simulink model "Simulare_cu_Ackermann"  (R2023b)
settings: Solver=VariableStepAuto  StartTime=0.0  StopTime=10  FixedStep=0.01  RelTol=1e-3
values from neighbouring files (symbols this model uses):
  K = Z/P    [LMI.m]    (also in Workspace.mat = 8.82782218537; model_simulation.m = lqr(A,B,Q,R,0.01))
  T = 0.8    [model_robust.m]
undefined symbols (not defined in the file or in its folder): L
settings Model: Creator=petri  LastModifiedBy=petri

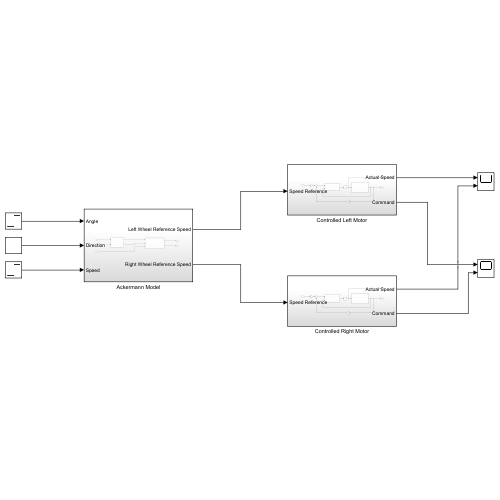
[thumbnail: Simulink's stored preview of the top-level diagram]
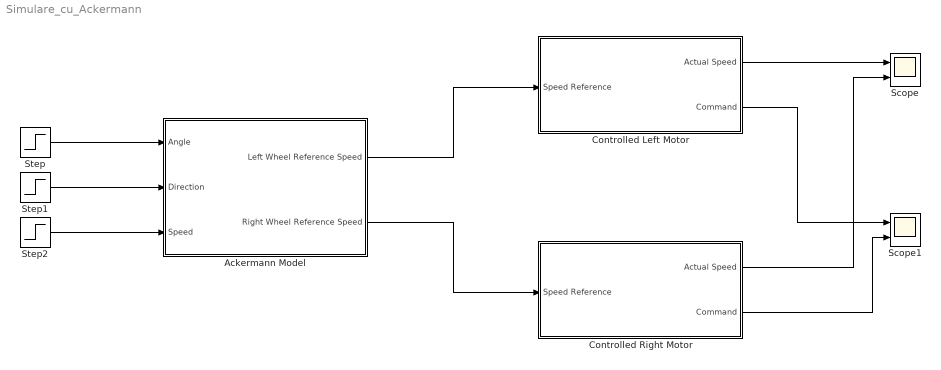
== system Simulare_cu_Ackermann ==
  Ackermann Model : Subsystem
  Controlled Left Motor : Subsystem
  Controlled Right Motor : Subsystem
  Scope : Scope  NumInputPorts=2
  Scope1 : Scope  NumInputPorts=2
  Step : Step  After=30  SampleTime=0
  Step1 : Step  SampleTime=0
  Step2 : Step  After=120  SampleTime=0
  wires:
  Ackermann Model/1(Left Wheel Reference Speed) -> Controlled Left Motor/1(Speed Reference)
  Ackermann Model/2(Right Wheel Reference Speed) -> Controlled Right Motor/1(Speed Reference)
  Step/1 -> Ackermann Model/1(Angle)
  Step1/1 -> Ackermann Model/2(Direction)
  Step2/1 -> Ackermann Model/3(Speed)
  Controlled Left Motor/1(Actual Speed) -> Scope/1
  Controlled Left Motor/2(Command) -> Scope1/1
  Controlled Right Motor/1(Actual Speed) -> Scope/2
  Controlled Right Motor/2(Command) -> Scope1/2

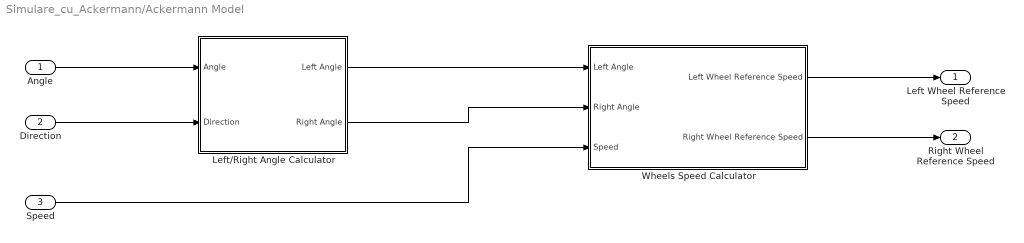
== system Simulare_cu_Ackermann/Ackermann Model ==
  Angle : Inport
  Direction : Inport  Port=2
  Speed : Inport  Port=3
  Left/Right Angle Calculator : Subsystem
  Wheels Speed Calculator : Subsystem
  Left Wheel Reference Speed : Outport
  Right Wheel Reference Speed : Outport  Port=2
  wires:
  Wheels Speed Calculator/1(Left Wheel Reference Speed) -> Left Wheel Reference Speed/1
  Left/Right Angle Calculator/2(Right Angle) -> Wheels Speed Calculator/2(Right Angle)
  Angle/1 -> Left/Right Angle Calculator/1(Angle)
  Left/Right Angle Calculator/1(Left Angle) -> Wheels Speed Calculator/1(Left Angle)
  Speed/1 -> Wheels Speed Calculator/3(Speed)
  Direction/1 -> Left/Right Angle Calculator/2(Direction)
  Wheels Speed Calculator/2(Right Wheel Reference Speed) -> Right Wheel Reference Speed/1

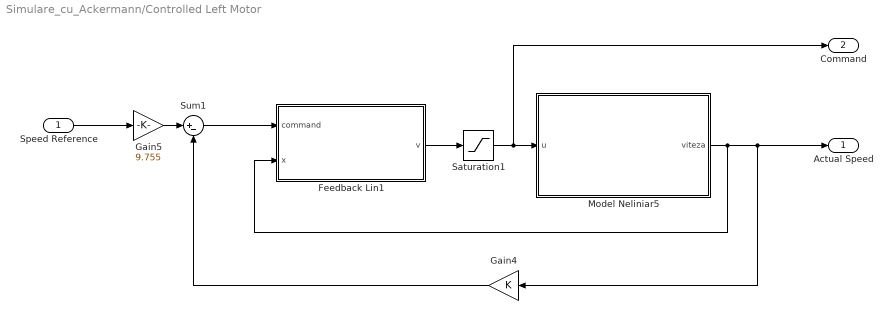
== system Simulare_cu_Ackermann/Controlled Left Motor ==
  Speed Reference : Inport
  Feedback Lin1 : Subsystem
  Gain4 : Gain  Gain=K
  Gain5 : Gain  Gain=9.755
  Model Neliniar5 : Subsystem
  Saturation1 : Saturate  UpperLimit=0.3  LowerLimit=0
  Sum1 : Sum  Inputs=|+-
  Actual Speed : Outport
  Command : Outport  Port=2
  wires:
  Speed Reference/1 -> Gain5/1
  Feedback Lin1/1(v) -> Saturation1/1
  Saturation1/1 -> Command/1, Model Neliniar5/1(u)
  Model Neliniar5/1(viteza) -> Actual Speed/1, Gain4/1, Feedback Lin1/2(x)
  Sum1/1 -> Feedback Lin1/1(command)
  Gain4/1 -> Sum1/2
  Gain5/1 -> Sum1/1

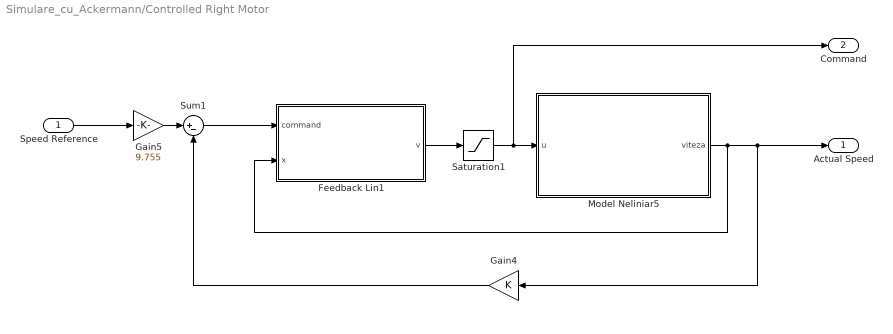
== system Simulare_cu_Ackermann/Controlled Right Motor ==
  Speed Reference : Inport
  Feedback Lin1 : Subsystem
  Gain4 : Gain  Gain=K
  Gain5 : Gain  Gain=9.755
  Model Neliniar5 : Subsystem
  Saturation1 : Saturate  UpperLimit=0.3  LowerLimit=0
  Sum1 : Sum  Inputs=|+-
  Actual Speed : Outport
  Command : Outport  Port=2
  wires:
  Speed Reference/1 -> Gain5/1
  Feedback Lin1/1(v) -> Saturation1/1
  Saturation1/1 -> Command/1, Model Neliniar5/1(u)
  Model Neliniar5/1(viteza) -> Actual Speed/1, Gain4/1, Feedback Lin1/2(x)
  Sum1/1 -> Feedback Lin1/1(command)
  Gain4/1 -> Sum1/2
  Gain5/1 -> Sum1/1

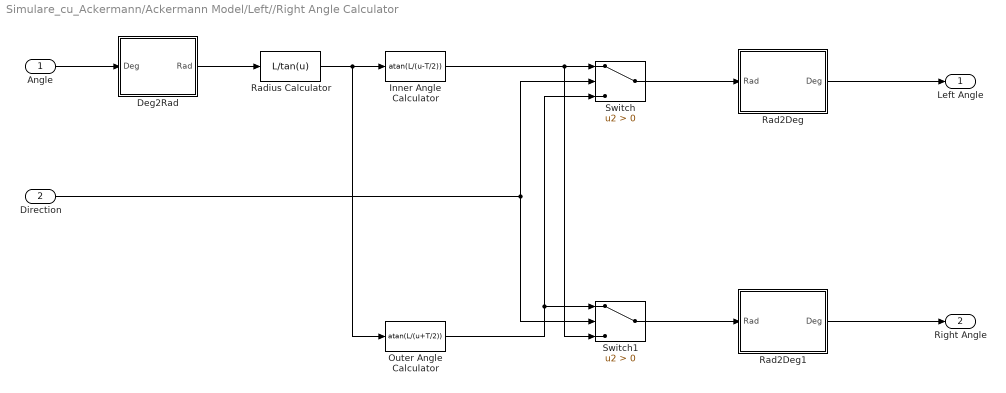
== system Simulare_cu_Ackermann/Ackermann Model/Left//Right Angle Calculator ==
  Angle : Inport
  Direction : Inport  Port=2
  Deg2Rad : Subsystem
  Inner Angle Calculator : Fcn  Expr=atan(L/(u-T/2))
  Outer Angle Calculator : Fcn  Expr=atan(L/(u+T/2))
  Rad2Deg : Subsystem
  Rad2Deg1 : Subsystem
  Radius Calculator : Fcn  Expr=L/tan(u)
  Switch : Switch  Criteria=u2 > Threshold  SaturateOnIntegerOverflow=off  InputSameDT=off
  Switch1 : Switch  Criteria=u2 > Threshold  SaturateOnIntegerOverflow=off  InputSameDT=off
  Left Angle : Outport
  Right Angle : Outport  Port=2
  wires:
  Direction/1 -> Switch/2, Switch1/2
  Angle/1 -> Deg2Rad/1(Deg)
  Outer Angle Calculator/1 -> Switch1/1, Switch/3
  Inner Angle Calculator/1 -> Switch/1, Switch1/3
  Switch/1 -> Rad2Deg/1(Rad)
  Switch1/1 -> Rad2Deg1/1(Rad)
  Rad2Deg1/1(Deg) -> Right Angle/1
  Rad2Deg/1(Deg) -> Left Angle/1
  Radius Calculator/1 -> Inner Angle Calculator/1, Outer Angle Calculator/1
  Deg2Rad/1(Rad) -> Radius Calculator/1

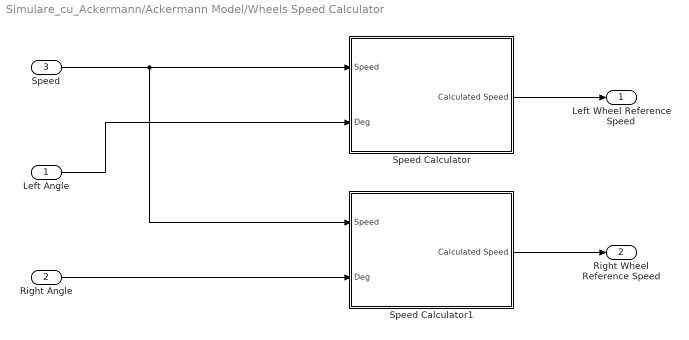
== system Simulare_cu_Ackermann/Ackermann Model/Wheels Speed Calculator ==
  Left Angle : Inport
  Right Angle : Inport  Port=2
  Speed : Inport  Port=3
  Speed Calculator : Subsystem
  Speed Calculator1 : Subsystem
  Left Wheel Reference Speed : Outport
  Right Wheel Reference Speed : Outport  Port=2
  wires:
  Speed Calculator1/1(Calculated Speed) -> Right Wheel Reference Speed/1
  Right Angle/1 -> Speed Calculator1/2(Deg)
  Speed/1 -> Speed Calculator/1(Speed), Speed Calculator1/1(Speed)
  Speed Calculator/1(Calculated Speed) -> Left Wheel Reference Speed/1
  Left Angle/1 -> Speed Calculator/2(Deg)

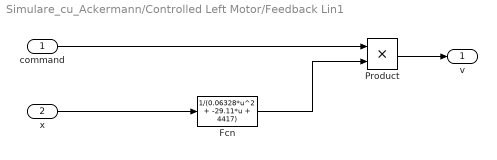
== system Simulare_cu_Ackermann/Controlled Left Motor/Feedback Lin1 ==
  command : Inport
  x : Inport  Port=2
  Fcn : Fcn  Expr=1/(0.06328*u^2 + -29.11*u + 4417)
  Product : Product
  v : Outport
  wires:
  Product/1 -> v/1
  Fcn/1 -> Product/2
  command/1 -> Product/1
  x/1 -> Fcn/1

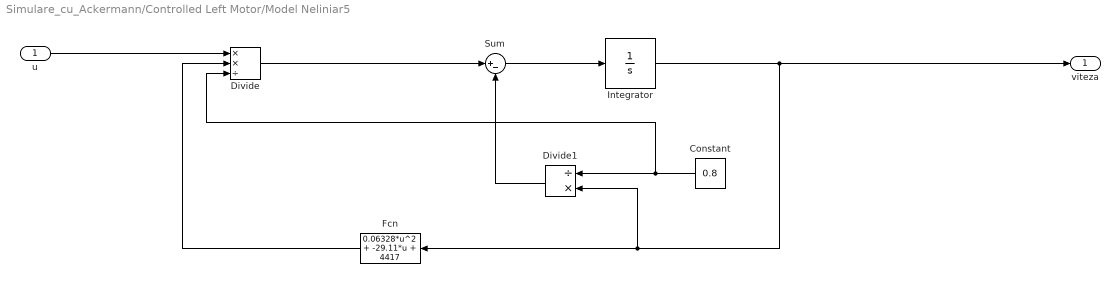
== system Simulare_cu_Ackermann/Controlled Left Motor/Model Neliniar5 ==
  u : Inport
  Constant : Constant  Value=0.8
  Divide : Product  Inputs=**/
  Divide1 : Product  Inputs=/*
  Fcn : Fcn  Expr=0.06328*u^2 + -29.11*u + 4417
  Integrator : Integrator
  Sum : Sum  Inputs=|+-
  viteza : Outport
  wires:
  u/1 -> Divide/1
  Constant/1 -> Divide1/1, Divide/3
  Integrator/1 -> viteza/1, Fcn/1, Divide1/2
  Sum/1 -> Integrator/1
  Divide1/1 -> Sum/2
  Divide/1 -> Sum/1
  Fcn/1 -> Divide/2

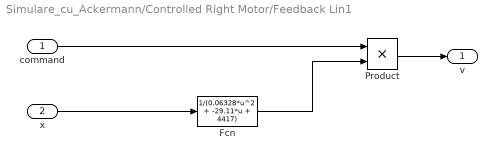
== system Simulare_cu_Ackermann/Controlled Right Motor/Feedback Lin1 ==
  command : Inport
  x : Inport  Port=2
  Fcn : Fcn  Expr=1/(0.06328*u^2 + -29.11*u + 4417)
  Product : Product
  v : Outport
  wires:
  Product/1 -> v/1
  Fcn/1 -> Product/2
  command/1 -> Product/1
  x/1 -> Fcn/1

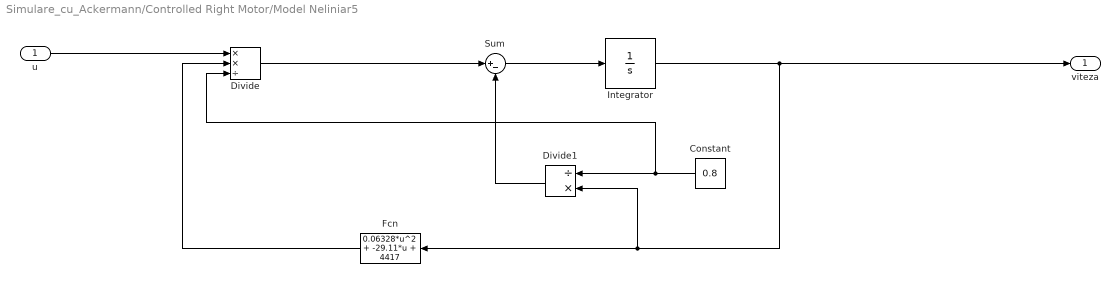
== system Simulare_cu_Ackermann/Controlled Right Motor/Model Neliniar5 ==
  u : Inport
  Constant : Constant  Value=0.8
  Divide : Product  Inputs=**/
  Divide1 : Product  Inputs=/*
  Fcn : Fcn  Expr=0.06328*u^2 + -29.11*u + 4417
  Integrator : Integrator
  Sum : Sum  Inputs=|+-
  viteza : Outport
  wires:
  u/1 -> Divide/1
  Constant/1 -> Divide1/1, Divide/3
  Integrator/1 -> viteza/1, Fcn/1, Divide1/2
  Sum/1 -> Integrator/1
  Divide1/1 -> Sum/2
  Divide/1 -> Sum/1
  Fcn/1 -> Divide/2

== system Simulare_cu_Ackermann/Ackermann Model/Left//Right Angle Calculator/Deg2Rad ==
  Deg : Inport
  Constant : Constant  Value=pi/180
  Product : Product
  Rad : Outport
  wires:
  Constant/1 -> Product/2
  Product/1 -> Rad/1
  Deg/1 -> Product/1

== system Simulare_cu_Ackermann/Ackermann Model/Left//Right Angle Calculator/Rad2Deg ==
  Rad : Inport
  Constant : Constant  Value=180/pi
  Product : Product
  Deg : Outport
  wires:
  Rad/1 -> Product/1
  Product/1 -> Deg/1
  Constant/1 -> Product/2

== system Simulare_cu_Ackermann/Ackermann Model/Left//Right Angle Calculator/Rad2Deg1 ==
  Rad : Inport
  Constant : Constant  Value=180/pi
  Product : Product
  Deg : Outport
  wires:
  Rad/1 -> Product/1
  Product/1 -> Deg/1
  Constant/1 -> Product/2

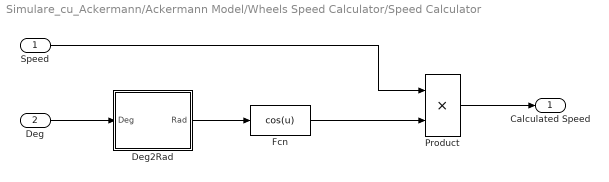
== system Simulare_cu_Ackermann/Ackermann Model/Wheels Speed Calculator/Speed Calculator ==
  Speed : Inport
  Deg : Inport  Port=2
  Deg2Rad : Subsystem
  Fcn : Fcn  Expr=cos(u)
  Product : Product
  Calculated Speed : Outport
  wires:
  Product/1 -> Calculated Speed/1
  Speed/1 -> Product/1
  Deg2Rad/1(Rad) -> Fcn/1
  Fcn/1 -> Product/2
  Deg/1 -> Deg2Rad/1(Deg)

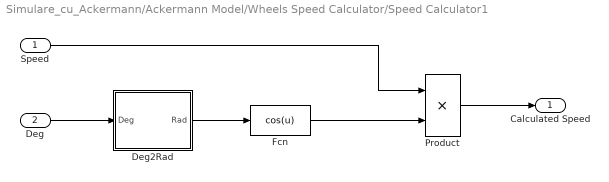
== system Simulare_cu_Ackermann/Ackermann Model/Wheels Speed Calculator/Speed Calculator1 ==
  Speed : Inport
  Deg : Inport  Port=2
  Deg2Rad : Subsystem
  Fcn : Fcn  Expr=cos(u)
  Product : Product
  Calculated Speed : Outport
  wires:
  Product/1 -> Calculated Speed/1
  Speed/1 -> Product/1
  Deg2Rad/1(Rad) -> Fcn/1
  Fcn/1 -> Product/2
  Deg/1 -> Deg2Rad/1(Deg)

== system Simulare_cu_Ackermann/Ackermann Model/Wheels Speed Calculator/Speed Calculator/Deg2Rad ==
  Deg : Inport
  Constant : Constant  Value=pi/180
  Product : Product
  Rad : Outport
  wires:
  Constant/1 -> Product/2
  Product/1 -> Rad/1
  Deg/1 -> Product/1

== system Simulare_cu_Ackermann/Ackermann Model/Wheels Speed Calculator/Speed Calculator1/Deg2Rad ==
  Deg : Inport
  Constant : Constant  Value=pi/180
  Product : Product
  Rad : Outport
  wires:
  Constant/1 -> Product/2
  Product/1 -> Rad/1
  Deg/1 -> Product/1
